simulink library "lib_hysteresis"  (R2023a)
settings: Solver=VariableStepAuto  StartTime=0.0  StopTime=10.0  RelTol=1e-3
undefined symbols (not defined in the file): lb_parInitOutp
settings Model: Creator=YXQ1WX  LastModifiedBy=xiaoqiang.yuan
settings OptimizationCC: ReuseModelBlockBuffer=off

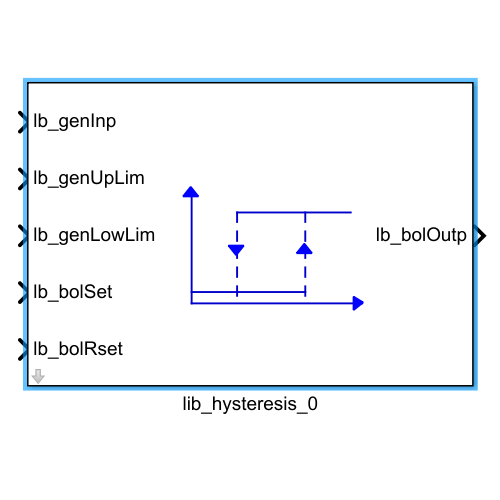
[thumbnail: Simulink's stored preview of the top-level diagram]
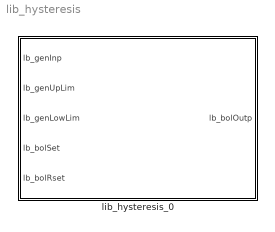
== system lib_hysteresis ==
  lib_hysteresis_0 : Subsystem  RTWFcnName=Hysteresis  RTWFileName=VHIT_control_library  mask(Hysteresis){}
      mask help:
      | 1. x(k) < xLo:           y(k) = yLo;
      | 2. xLo ≤ x(k) ≤ xHi:   y(k) = y(k-1);
      | 3. x(k) > xHi:           y(k) = yHi.
      settings: RTWFcnNameOpts=User specified
      mask DialogControl DescGroupVar Prompt: VHIT control library
      mask DialogControl DescTextVar Prompt: For Hysteresis
      mask Display:
      | color('Blue')
      | fac = 1.2;
      | o_x = 72;
      | o_y = 36;
      | o_hi = 50;
      | o_len = 75;
      | plot([o_x,o_x,o_x+o_len]*fac, [o_y+o_hi,o_y,o_y]*fac);
      | patch([o_x-3,o_x+3,o_x,o_x-3]*fac, [o_y+o_hi-3,o_y+o_hi-3,o_y+o_hi+1,o_y+o_hi-3]*fac,[0,0,1])
      | patch([o_x+o_len-3,o_x+o_len-3,o_x+o_len+1,o_x+o_len-3]*fac, [o_y+3,o_y-3,o_y,o_y+3]*fac,[0,0,1])
      | color('Blue')
      | plot(([0,50]+o_x)*fac, ([5,5]+o_y)*fac);
      | plot(([20,70]+o_x)*fac, ([40,40]+o_y)*fac);
      | for i = 1:5
      |     plot([20+o_x,20+o_x]*fac, [o_y+(2*i-1)*4,o_y+2*i*4]*fac);
      | end
      | for i = 1:5
      |     plot([50+o_x,50+o_x]*fac, [o_y+(2*i-1)*4,o_y+2*i*4]*fac);
      | end
      | patch([o_x+50-3,o_x+50+3,o_x+50,o_x+50-3]*fac, [o_y+25-3,o_y+25-3,o_y+25+1,o_y+25-3]*fac,[0,0,1]);
      | patch([o_x+20-3,o_x+20+3,o_x+20,o_x+20-3]*fac, [o_y+22+3,o_y+22+3,o_y+22-1,o_y+22+3]*fac,[0,0,1]);
      | color('Black');
      | port_label('output', 1, 'lb_bolOutp');
      | port_label('input', 1, 'lb_genInp');
      | port_label('input', 2, 'lb_genUpLim');
      | port_label('input', 3, 'lb_genLowLim');
      | port_label('input', 4, 'lb_bolSet');
      | port_label('input', 5, 'lb_bolRset');

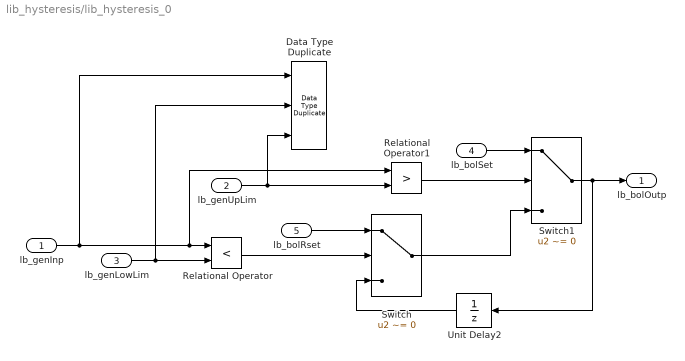
== system lib_hysteresis/lib_hysteresis_0 ==
  lb_genInp : Inport
  lb_genUpLim : Inport  Port=2
  lb_genLowLim : Inport  Port=3
  lb_bolSet : Inport  Port=4
  lb_bolRset : Inport  Port=5
  Data Type Duplicate : DataTypeDuplicate  NumInputPorts=3
  Relational Operator : RelationalOperator  Operator=<  OutDataTypeStr=boolean  InputSameDT=off
  Relational Operator1 : RelationalOperator  Operator=>  OutDataTypeStr=boolean  InputSameDT=off
  Switch : Switch  Criteria=u2 ~= 0  SaturateOnIntegerOverflow=off  InputSameDT=off  OutDataTypeStr=Inherit: Same as first input
  Switch1 : Switch  Criteria=u2 ~= 0  SaturateOnIntegerOverflow=off  InputSameDT=off  OutDataTypeStr=Inherit: Same as first input
  Unit Delay2 : UnitDelay  InitialCondition=lb_parInitOutp  SampleTime=-1  HasFrameUpgradeWarning=on
  lb_bolOutp : Outport
  wires:
  Switch/1 -> Switch1/3
  Relational Operator1/1 -> Switch1/2
  Relational Operator/1 -> Switch/2
  lb_bolRset/1 -> Switch/1
  lb_bolSet/1 -> Switch1/1
  lb_genLowLim/1 -> Data Type Duplicate/2, Relational Operator/2
  lb_genInp/1 -> Data Type Duplicate/1, Relational Operator1/1, Relational Operator/1
  Unit Delay2/1 -> Switch/3
  Switch1/1 -> Unit Delay2/1, lb_bolOutp/1
  lb_genUpLim/1 -> Data Type Duplicate/3, Relational Operator1/2
